simulink model "exp2_ref版"  (R2024b)
settings: Solver=FixedStepAuto  StartTime=0.0  StopTime=0.1  FixedStep=0.0001  RelTol=1e-3
values from neighbouring files (symbols this model uses):
  harmonics_filters = filter_b(f, Nh)    [untitled.m]
undefined symbols (not defined in the file or in its folder): den_dc, num_dc
settings Model: Creator=86195  LastModifiedBy=86195

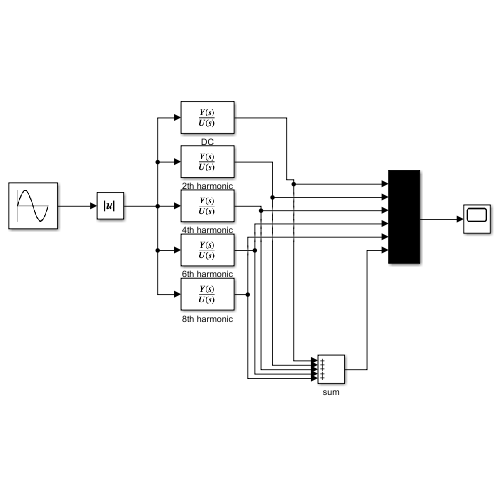
[thumbnail: Simulink's stored preview of the top-level diagram]
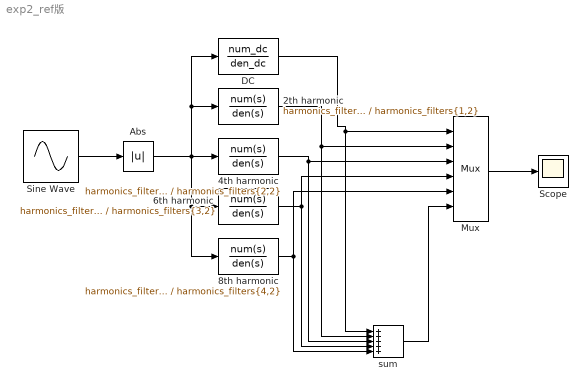
== system exp2_ref版 ==
  2th harmonic : TransferFcn  Numerator=harmonics_filters{1,1}  Denominator=harmonics_filters{1,2}
  4th harmonic : TransferFcn  Numerator=harmonics_filters{2,1}  Denominator=harmonics_filters{2,2}
  6th harmonic : TransferFcn  Numerator=harmonics_filters{3,1}  Denominator=harmonics_filters{3,2}
  8th harmonic : TransferFcn  Numerator=harmonics_filters{4,1}  Denominator=harmonics_filters{4,2}
  Abs : Abs  SaturateOnIntegerOverflow=off
  DC : TransferFcn  Numerator=num_dc  Denominator=den_dc
  Mux : Mux  Inputs=6
  Scope : Scope
  Sine Wave : Sin  Amplitude=10  Frequency=100*2*pi  Phase=pi/2  SampleTime=0
  sum : Sum  Inputs=+++++
  wires:
  Sine Wave/1 -> Abs/1
  Abs/1 -> 8th harmonic/1, 6th harmonic/1, 4th harmonic/1, DC/1, 2th harmonic/1
  DC/1 -> sum/1, Mux/1
  2th harmonic/1 -> sum/2, Mux/2
  4th harmonic/1 -> sum/3, Mux/3
  6th harmonic/1 -> sum/4, Mux/4
  8th harmonic/1 -> sum/5, Mux/5
  Mux/1 -> Scope/1
  sum/1 -> Mux/6
